simulink model "UDPtest"  (R2024b)
settings: Solver=FixedStepAuto  StartTime=0.0  StopTime=inf  RelTol=1e-3
values from neighbouring files (symbols this model uses):
  C = [1 0 0 0; 0 1 0 0]    [Car_test_UDP.m]    (also in Final_Code_GPS.m; Final_Code_plotting_reset_kalman.m; KalmanFilter.m)
undefined symbols (not defined in the file or in its folder): f
libraries: sim3dautolib x2, sim3dlib x1, instrumentlib x1
settings Model: Creator=ritvi  LastModifiedBy=ritvi

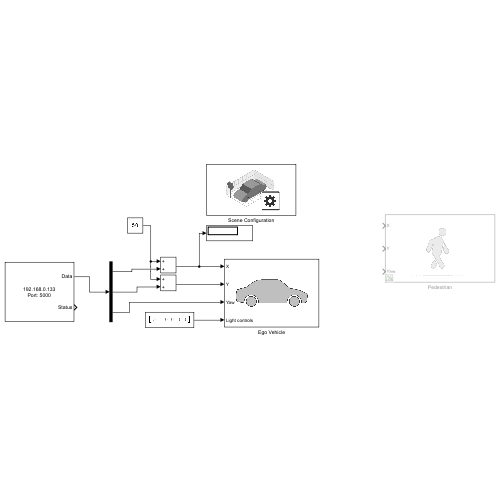
[thumbnail: Simulink's stored preview of the top-level diagram]
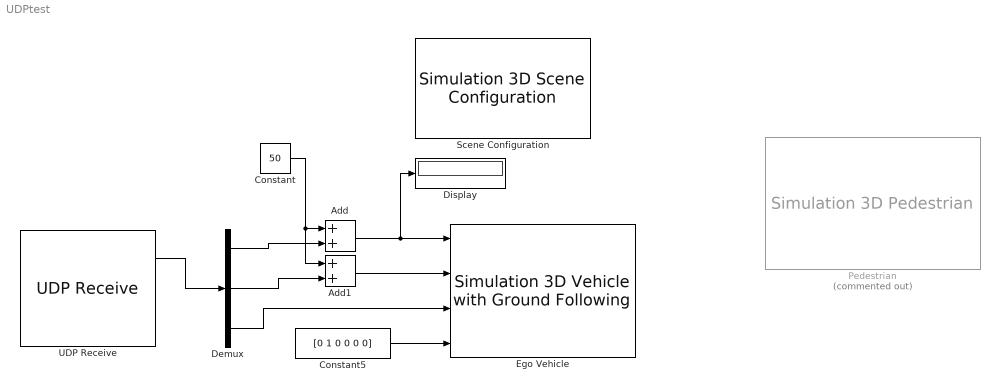
== system UDPtest ==
  Add : Sum
  Add1 : Sum
  Constant : Constant  Value=50
  Constant5 : Constant  Value=[0 1 0 0 0 0]
  Demux : Demux  Outputs=3
  Display : Display
  Ego Vehicle : sim3dautolib/Simulation 3D Vehicle with Ground Following  Priority=-1  PassVehMesh=Hatchback  MeshPath=/MathWorksSimulation/Vehicles/Muscle/Meshes/SK_MuscleCar.SK_MuscleCar  TrackWidth=1.9  WheelBase=3  WheelRadius=0.35  VehColor=Red  InitialPos=[50, 50, 0]  InitialRot=[0, 0, 90]  ActorName=SimulinkVehicle1  SampleTime=-1  ActorType=SimulinkVehicle  ID=1  aMode=3  ActorTag=SimulinkVehicle1  CoordinateScheme=ISO  VehLightsControl=on  HeadlightColor=[ 1, 1, 1 ]  HighBeamIntensity=100000  LowBeamIntensity=60000  HighBeamConeAngle=70  LowBeamConeAngle=70  LeftHeadlightOrientation=[ 0, 0 ]  RightHeadlightOrientation=[ 0, 0 ]  BrakelightIntensity=500  ReverselightIntensity=500  SignallightIntensity=500  SignallightPeriod=1  SignalPulseWidth=50  TransformOutportEnabled=off
      settings: LibrarySourceBlock=drivingsim3d/Simulation 3D Vehicle with Ground Following
  Pedestrian : sim3dautolib/Simulation 3D Pedestrian  Priority=-1  Commented=on  PedestrianType=Female 1  Scale=[1, 1, 1]  InitialPos=[0, 0, 0]  InitialYaw=0  ActorName=SimulinkPedestrian1  SampleTime=-1  ActorType=SimulinkPedestrian  ActorTag=SimulinkPedestrian1  ID=1  aMode=3  CoordinateScheme=ISO  TransformOutportEnabled=off
      settings: LibrarySourceBlock=drivingsim3d/Simulation 3D Pedestrian
  Scene Configuration : sim3dlib/Simulation 3D Scene Configuration  Priority=0  ProjectFormat=Unreal Editor  SceneDesc=Large parking lot  ProjectName=C:\Program Files\MATLAB\R2024b\toolbox\shared\sim3d_projects\automotive_project_windows\UE\WindowsNoEditor\VehicleSimulation.exe  ScenePath=/Game/Maps/HwStrght  UEProjPath=C:\Local\AutoVrtlEnv\AutoVrtlEnv.uproject  EnableOpenDRIVE=off  vehTagList={'Custom';'Scene Origin';'SimulinkVehicle1'}  vehTag=SimulinkVehicle1  FreeCameraInitialTranslation=[0, 0, 0]  FreeCameraDefaultInitialTranslation=[-6, 0, 2]  FreeCameraInitialRotation=[0, 0, 0]  FreeCameraDefaultInitialRotation=[0, -15, 0]  OpVisEn=off  Ts=0.05  EnableWindow=on  EnableRemoteAccess=off  EnableWeather=off  SunAzimuth=183.600  SunAltitude=0.0  EnableGeospatialSun=off  Latitude=0  Longitude=0  Date=2023-01-01  Time=10:30:00  GeoTimeZone=-5.0  SunDaylightSaving=off  wind=1  clouds=50.0  EnableVolumetricClouds=off  CloudCoverage=0  CloudAltitude=6  fog=0.0  rain=18.0  RaindropsEffect=off  SnowDensity=0  EnableGeospatial=off  UseTrueOrigin=off  OriginHeight=200  OriginLatitude=40.744652  OriginLongitude=-73.988864  MapStyle=Aerial  AdditionalAssetIDs=[]  UseAdvancedSunSky=off  SolarTime=11  TimeZone=-5  Day=21  Month=9  Year=2022  UseDaylightSavingTime=on  DSTStartDay=10  DSTStartMonth=3  DSTEndDay=3  DSTEndMonth=11  DSTSwitchHour=2  sensorTag=MainCamera1  sensorId=1  sensorName=MainCamera1  mountLoc=Origin  offsetFlag=off  tmountOffset=[0, 0, 0]  rmountOffset=[0, 0, 0]  HorizontalResolution=1280  VerticalResolution=720  HorizontalFOV=60  mountPoint=[0 0 0]  mountOrientation=[0 0 0]  aMode=3  ID=1  GeoTrigger=Inactive
      settings: LibrarySourceBlock=drivingsim3d/Simulation 3D Scene Configuration
  UDP Receive : instrumentlib/UDP Receive  LocalAddress=192.168.0.133  LocalPort=5000  EnablePortSharing=off  Host=localhost  Port=9090  GetLatestData=on  DataSize=[ 1, 3 ]  DataType=double  ASCIIFormatting=%f,  Terminator=LF  CustomTerminator=10  ByteOrder=big-endian  EnableBlockingMode=off  Timeout=10  SampleTime=0.01  SimulateUsing=Interpreted execution
  wires:
  Constant5/1 -> Ego Vehicle/4
  UDP Receive/1 -> Demux/1
  Demux/3 -> Ego Vehicle/3
  Demux/2 -> Add1/2
  Demux/1 -> Add/2
  Constant/1 -> Add1/1, Add/1
  Add/1 -> Display/1, Ego Vehicle/1
  Add1/1 -> Ego Vehicle/2
